simulink model "StatefulLSTMPyTorchExportedProgram"  (R2026a)
settings: Solver=VariableStepAuto  StopTime=16.5
undefined symbols (not defined in the file or in its folder): float32
libraries: dlosslib x1, pycoexlib x1
settings Model: Creator=hravisha  LastModifiedBy=hravisha

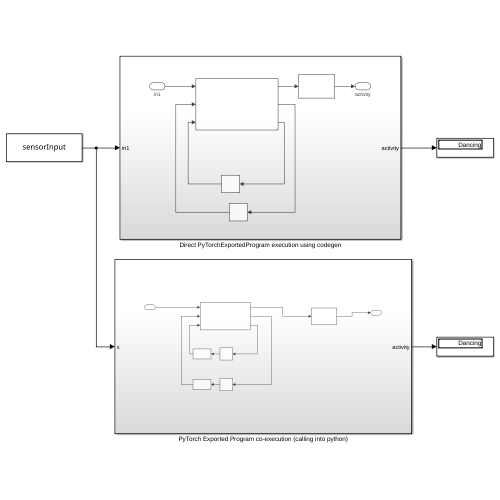
[thumbnail: Simulink's stored preview of the top-level diagram]
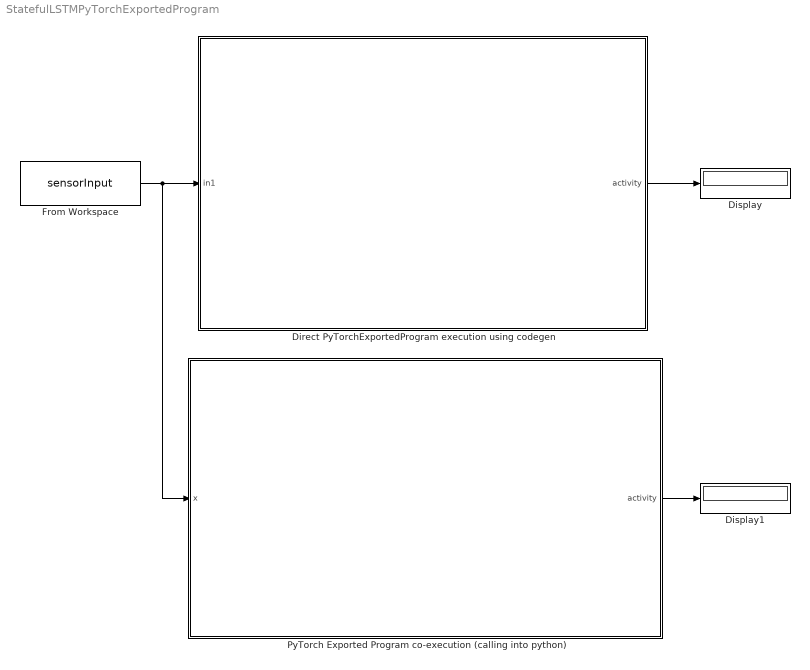
== system StatefulLSTMPyTorchExportedProgram ==
  Direct PyTorchExportedProgram execution using codegen : Subsystem
  Display : Display
  Display1 : Display
  From Workspace : FromWorkspace  VariableName=sensorInput  SampleTime=1.5
  PyTorch Exported Program co-execution (calling into python) : Subsystem
  wires:
  PyTorch Exported Program co-execution (calling into python)/1(activity) -> Display1/1
  Direct PyTorchExportedProgram execution using codegen/1(activity) -> Display/1
  From Workspace/1 -> PyTorch Exported Program co-execution (calling into python)/1(x), Direct PyTorchExportedProgram execution using codegen/1(in1)

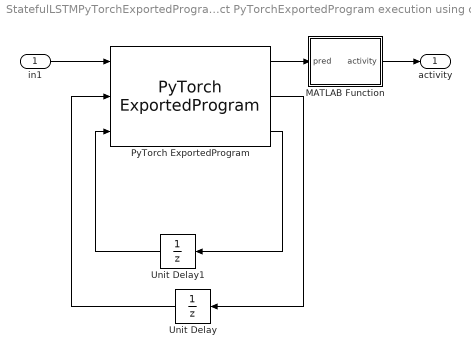
== system StatefulLSTMPyTorchExportedProgram/Direct PyTorchExportedProgram execution using codegen ==
  in1 : Inport
  MATLAB Function : MATLAB Function  TreatAsAtomicUnit=on
  PyTorch ExportedProgram : dlosslib/PyTorch ExportedProgram  ModelFilePath=/local-ssd/hravisha/directCodegenLectureSeminar/matlab_demo/stateful_lstm.pt2  SampleTime=-1  InputsTable={ 'in1', 'single', '[1 75 3]', '[1 2 3]'; 'in2', 'single', '[1 1 50]', '[1 2 3]'; 'in3', 'single', '[1 1 50]', '[1 2 3]' }  OutputsTable={ 'out1', 'single', '[1 75 5]', '[1 75 5]', '[1 2 3]'; 'out2', 'single', '[1 1 50]', '[1 1 50]', '[1 2 3]'; 'out3', 'single', '[1 1 50]', '[1 1 50]', '[1 2 3]' }  LastKnownModelFilePath=/local-ssd/hravisha/directCodegenLectureSeminar/matlab_demo/stateful_lstm.pt2  LastKnownModelTimeStamp=740076.3848379629  LastKnownFcnName=<empty>
  Unit Delay : UnitDelay  InitialCondition=zeros(1,1,50,'single')  SampleTime=-1
  Unit Delay1 : UnitDelay  InitialCondition=zeros(1,1,50,'single')  SampleTime=-1
  activity : Outport
  wires:
  MATLAB Function/1(activity) -> activity/1
  PyTorch ExportedProgram/3 -> Unit Delay1/1
  PyTorch ExportedProgram/2 -> Unit Delay/1
  PyTorch ExportedProgram/1 -> MATLAB Function/1(pred)
  in1/1 -> PyTorch ExportedProgram/1
  Unit Delay1/1 -> PyTorch ExportedProgram/3
  Unit Delay/1 -> PyTorch ExportedProgram/2

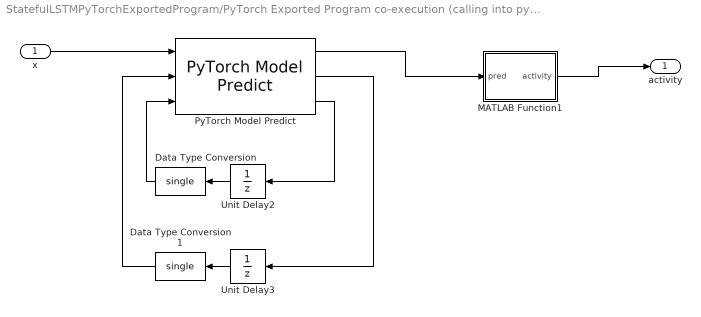
== system StatefulLSTMPyTorchExportedProgram/PyTorch Exported Program co-execution (calling into python) ==
  x : Inport
  Data Type Conversion : DataTypeConversion  OutDataTypeStr=single  SaturateOnIntegerOverflow=off  RndMeth=Floor
  Data Type Conversion1 : DataTypeConversion  OutDataTypeStr=single  SaturateOnIntegerOverflow=off  RndMeth=Floor
  MATLAB Function1 : MATLAB Function  TreatAsAtomicUnit=on
  PyTorch Model Predict : pycoexlib/PyTorch Model Predict  ModelFile=/local-ssd/hravisha/directCodegenLectureSeminar/matlab_demo/stateful_lstm.pt2  IsWeightFile=off  DeviceComboBox=cpu  InputTable={'x','float32','[1 2 3]','3';'h_0','float32','[1 2 3]','3';'c_0','float32','[1 2 3]','3'}  OutputTable={'linear','[1 2 3]','';'getitem_1','[1 2 3]','';'getitem_2','[1 2 3]',''}  SampleTime=-1  Device=cpu  InputDatatypes=float32,float32,float32  InputNumDims=3,3,3  InputPermutations=[1 2 3],[1 2 3],[1 2 3]  OutputPermutations=[1 2 3],[1 2 3],[1 2 3]  PythonCoexecutionBlockType=PyTorchModelBlock  VariableOutputMaxSizes=[],[],[]  InspectorCache=<binary blob, 7960 chars, not shown>
  Unit Delay2 : UnitDelay  InitialCondition=zeros(1,1,50,'single')  SampleTime=-1
  Unit Delay3 : UnitDelay  InitialCondition=zeros(1,1,50,'single')  SampleTime=-1
  activity : Outport
  wires:
  Unit Delay2/1 -> Data Type Conversion/1
  Data Type Conversion1/1 -> PyTorch Model Predict/2
  Unit Delay3/1 -> Data Type Conversion1/1
  PyTorch Model Predict/1 -> MATLAB Function1/1(pred)
  x/1 -> PyTorch Model Predict/1
  Data Type Conversion/1 -> PyTorch Model Predict/3
  PyTorch Model Predict/3 -> Unit Delay2/1
  PyTorch Model Predict/2 -> Unit Delay3/1
  MATLAB Function1/1(activity) -> activity/1

== matlab function StatefulLSTMPyTorchExportedProgram/PyTorch Exported Program co-execution (calling into python)/MATLAB Function1 ==
  data: pred input; activity output
function activity = classifyActivity(pred)
    % pred is [1, 75, 5] — take last timestep, find argmax
    lastStep = pred(1, end, :);       % [1, 1, 5]
    scores = squeeze(lastStep);        % [5, 1]
    [~, idx] = max(scores);
    activity = ActivityLabel(idx);
end

== matlab function StatefulLSTMPyTorchExportedProgram/Direct PyTorchExportedProgram execution using codegen/MATLAB Function ==
  data: pred input; activity output
function activity = classifyActivity(pred)
    % pred is [1, 75, 5] — take last timestep, find argmax
    lastStep = pred(1, end, :);       % [1, 1, 5]
    scores = squeeze(lastStep);        % [5, 1]
    [~, idx] = max(scores);
    activity = ActivityLabel(idx);
end
